simulink model "test"  (R2022a)
settings: Solver=VariableStepAuto  StartTime=0.0  StopTime=10.0  RelTol=1e-3
settings Model: Creator=q541028  LastModifiedBy=q541028

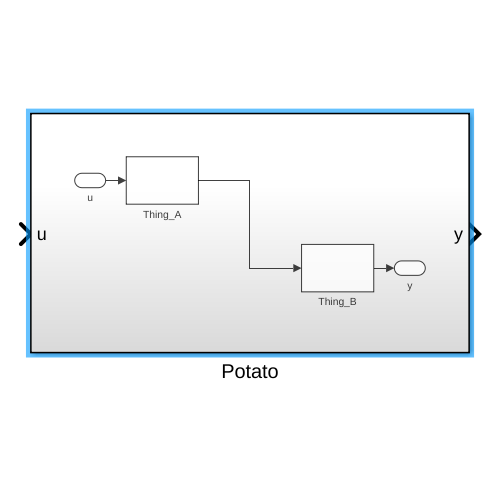
[thumbnail: Simulink's stored preview of the top-level diagram]
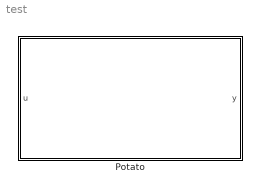
== system test ==
  Potato : Subsystem

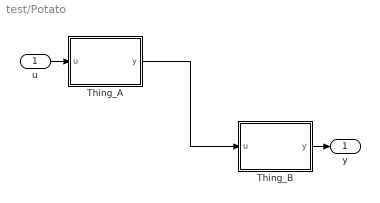
== system test/Potato ==
  u : Inport
  Thing_A : MATLAB Function  TreatAsAtomicUnit=on
  Thing_B : MATLAB Function  TreatAsAtomicUnit=on
  y : Outport
  wires:
  Thing_A/1(y) -> Thing_B/1(u)
  Thing_B/1(y) -> y/1
  u/1 -> Thing_A/1(u)

== matlab function test/Potato/Thing_A ==
  data: u input; y output
function y = fcn(u)

y = u;

== matlab function test/Potato/Thing_B ==
  data: u input; y output
function y = fcn(u)
%| pragma Tag("foo.bar");
y = u;
